simulink model "CML_Effort_Reward_Mapping"  (R2015a)
settings: Solver=ode4  SolverMode=MultiTasking  StartTime=0.0  StopTime=inf  FixedStep=BKIN_STEP_TIME  RelTol=1e-3
StartFcn:
  |  warndlg('Dexterit-E models cannot run under simulation. Please compile your model and run it from within Dexterit-E.');set_param(bdroot,'SimulationCommand','stop')
model workspace (MAT data in the model file):
  BKIN_STEP_TIME = 0.00025
  col_x = 1
  col_y = 2
  VRAD = 3
  COLOR = 4
  TARGET_COL = 2
  BKIN_KINEMATIC_FRAME_SIZE = 400
  E_NO_EVENT = 0
  K_START_TGT = 1
  INIT_DUR = 6
  TP_ITI = 10
  K_JOINT_ASSESSED = 2
  TEXT1 = 6
  TEXT2 = 7
  HEIGHT = 9
  STROKE_WIDTH = 10
  GOAL_F_PCT = 3
  DO_FDBK = 9
  MAX_MOVE_TIME = 8
  MIN_FORCE = 5
  E_TEST_MVC = 1
  E_HOLD_MVC = 3
  E_EOT = 10
  E_FORCE_TRIAL = 11
  E_HOLD_FORCE = 13
  K_BAR_TGT = 3
  K_MVC_TEXT_TGT = 5
  E_INIT_FORCE = 12
  E_SET_MVC = 2
  K_MVC = 6
  COLOR_SEL = 5
  ROTATION = 12
  K_RWD_TGT = 4
  E_ACCEPT_MVC = 5
  ACCEPT_MVC = 2
  REJECT_MVC = 3
  TEXT3 = 8
  REWARD_VAL = 4
  HOLD_TIME = 7
  E_REPORT_TRIAL = 21
  E_REPORT_RESPONSE = 22
  E_WAIT_JS_THRESH = 23
  E_AT_JS_THRESH = 24
  E_WAIT_JS = 27
  THEIGHT = 11
  TRIAL_TYPE = 1
  E_CHECK_MVC = 4
  E_REJECT_MVC = 6
  E_TRIAL_ACCEPTED = 25
  E_TRIAL_REJECTED = 26
undefined symbols (not defined in the file): magnitude
libraries: simulink x10, Video x9, slrtlib x8, General x3, KINARM_IO x2, KINARM_loads x2, KINARM_general x1, xpcnilib x1
(part 1 of 2)
CloseFcn:
  | rtwprivate ssgencode ModelCloseRequest b2lab2d
settings Model: ModifiedComment=chris -- Wed Feb 16 09:18:30 2005 -- Version 1.1384  ExtModeArmWhenConnect=off  ExtModeLogAll=off  LastModifiedBy=User
settings SolverCC: EnableConcurrentExecution=on  AutoInsertRateTranBlk=on
settings DataIOCC: LimitDataPoints=off  SignalLoggingSaveFormat=ModelDataLogs  SaveOutput=off  SaveTime=off  SignalLoggingName=sigsOut
settings OptimizationCC: BlockReduction=off  BooleanDataType=off  OptimizeBlockIOStorage=off  BufferReuse=off  GlobalBufferReuse=off  ExpressionFolding=off  ExpressionDepthLimit=2147483647  LocalBlockOutputs=off  InitFltsAndDblsToZero=on
settings DebuggingCC: SaveWithParameterizedLinksMsg=none  UnderspecifiedInitializationDetection=Classic  MergeDetectMultiDrivingBlocksExec=none  SignalResolutionControl=TryResolveAllWithWarning  MultiTaskDSMMsg=warning  FcnCallInpInsideContextMsg=UseLocalSettings  StateNameClashWarn=warning  StrictBusMsg=ErrorOnBusTreatedAsVector
settings HardwareCC: ProdIntDivRoundTo=Zero  ProdEndianess=LittleEndian  ProdLongLongMode=on  ProdHWDeviceType=Generic->32-bit x86 compatible  TargetHWDeviceType=32-bit Generic
settings SFSimCC: SimParseCustomCode=off
settings RTWCC: SystemTargetFile=slrt.tlc  TemplateMakefile=slrt_default_tmf  Description=Simulink Real-Time  RTWCompilerOptimization=on
settings CodeAppCC: MaxIdLength=63
settings SimulinkRealTimeCC: TargetFcnLib=ansi_tfl_tmw.mat  GeneratePreprocessorConditionals=Disable all  xPCisDownloadable=off

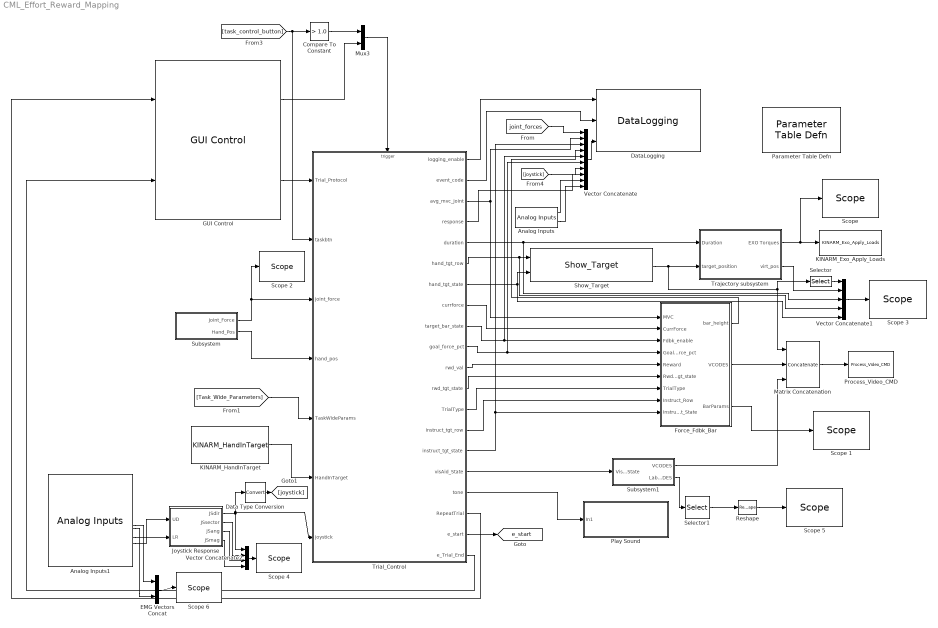
== system CML_Effort_Reward_Mapping ==
  Analog Inputs : KINARM_IO/Analog Inputs  channel=[18,19]  range=[5]  coupling=[0]  scantime6071e=1.28e-5  scantime6229=5e-6  sampletime=0.001  slot=-1  oscantime6071e=0
  Analog Inputs1 : KINARM_IO/Analog Inputs  channel=[1:32]  range=[5, 5, 5, 5, 5, 5, 5, 5,5, 5, 5, 5, 5, 5, 5, 5,5, 5, 5, 5, 5, 5, 5, 5,5, 5, 5, 5, 5, 5, 5, 5,]  coupling=[0, 0, 0, 0, 0, 0, 0, 0,0, 0, 0, 0, 0, 0, 0, 0,0, 0, 0, 0, 0, 0, 0, 0,0, 0, 0, 0, 0, 0, 0, 0,]  scantime6071e=1.28e-5  scantime6229=5e-6  sampletime=0.001  slot=-1  oscantime6071e=0
  Compare To Constant : simulink/Logic and Bit Operations/Compare To Constant  relop=>  const=1.0  OutDataTypeStr=boolean
  Data Type Conversion : DataTypeConversion
  DataLogging : General/DataLogging  log_event_codes=on  log_analog_inputs=on  show_time_remaining=off  ecat_include=on
      link override Poll KINARM/EPTorqueCMD: GotoTag=KINARMEPTorqueCMD
      link override Poll KINARM/TorqueCMD: GotoTag=KINARMTorqueCMD
  EMG Vectors Concat : Concatenate
  Force_Fdbk_Bar : Subsystem
  GUI Control : General/GUI Control  task_version=1.0  show_repeat_trial_flag=on  use_custom_tp=off  target_type_str=Circle  Target_Type=1  XYcols=[1 2]  Vcols=3  Lcols=4  indices_padding=[0 0 0 0;0 0 0 0]  target_table_rows=64  load_table_rows=20  tp_table_rows=100
  Joystick Response : Subsystem
  KINARM_Exo_Apply_Loads : KINARM_loads/KINARM_Exo_Apply_Loads  up_duration=1000  down_duration=1000  max_torque=10  limit_motors=off
  KINARM_HandInTarget : KINARM_general/KINARM_HandInTarget  use_dominant_hand=on  target_type=Circle  num_states=1  attribcol1=[VRAD]  attribcol2=[0]  attribcol3=[0]  attribcol4=[0]  attribcol5=[0]
  Matrix Concatenation : Concatenate  NumInputs=3  Mode=Multidimensional array
  Mux3 : Mux  Inputs=2
  Parameter Table Defn : General/Parameter Table Defn  ShowInLibBrowser=0
  Play Sound : Subsystem
  Process_Video_CMD : Video/Process_Video_CMD  video_delay=0
  Reshape : Reshape
  "Scope " : slrtlib/Displays and Logging/Scope   scopeno=6  scopetype=Target  autostart=on  viewmode=Numerical  formatstr='%15.6f'  grid=on  ylimits=[0,0]  nosamples=250  noprepostsamples=0  interleave=1  triggermode=FreeRun  triggersignal=1  trigsignalfromport=off  triggerlevel=0.0  triggerslope=Either  triggerscope=1  triggersample=0  filename=data.dat  mode=Lazy  writesize=512  autorestart=off  dynamicfilemode=off  maxwritefilesize=512*1024^2
  Scope 1 : slrtlib/Displays and Logging/Scope   scopeno=2  scopetype=Target  autostart=on  viewmode=Numerical  formatstr='%15.6f'  grid=on  ylimits=[0,0]  nosamples=250  noprepostsamples=0  interleave=1  triggermode=FreeRun  triggersignal=1  trigsignalfromport=off  triggerlevel=0.0  triggerslope=Either  triggerscope=1  triggersample=0  filename=data.dat  mode=Lazy  writesize=512  autorestart=off  dynamicfilemode=off  maxwritefilesize=512*1024^2
  Scope 2 : slrtlib/Displays and Logging/Scope   scopeno=3  scopetype=Target  autostart=on  viewmode=Numerical  formatstr='%15.6f'  grid=on  ylimits=[0,0]  nosamples=250  noprepostsamples=0  interleave=1  triggermode=FreeRun  triggersignal=1  trigsignalfromport=off  triggerlevel=0.0  triggerslope=Either  triggerscope=1  triggersample=0  filename=data.dat  mode=Lazy  writesize=512  autorestart=off  dynamicfilemode=off  maxwritefilesize=512*1024^2
  Scope 3 : slrtlib/Displays and Logging/Scope   scopeno=5  scopetype=Target  autostart=on  viewmode=Numerical  formatstr='%15.6f'  grid=on  ylimits=[0,0]  nosamples=250  noprepostsamples=0  interleave=1  triggermode=FreeRun  triggersignal=1  trigsignalfromport=off  triggerlevel=0.0  triggerslope=Either  triggerscope=1  triggersample=0  filename=data.dat  mode=Lazy  writesize=512  autorestart=off  dynamicfilemode=off  maxwritefilesize=512*1024^2
  Scope 4 : slrtlib/Displays and Logging/Scope   scopeno=1  scopetype=Target  autostart=on  viewmode=Numerical  formatstr='%15.6f'  grid=on  ylimits=[0,0]  nosamples=250  noprepostsamples=0  interleave=1  triggermode=FreeRun  triggersignal=1  trigsignalfromport=off  triggerlevel=0.0  triggerslope=Either  triggerscope=1  triggersample=0  filename=data.dat  mode=Lazy  writesize=512  autorestart=off  dynamicfilemode=off  maxwritefilesize=512*1024^2
  Scope 5 : slrtlib/Displays and Logging/Scope   scopeno=7  scopetype=Target  autostart=on  viewmode=Numerical  formatstr='%15.6f'  grid=on  ylimits=[0,0]  nosamples=250  noprepostsamples=0  interleave=1  triggermode=FreeRun  triggersignal=1  trigsignalfromport=off  triggerlevel=0.0  triggerslope=Either  triggerscope=1  triggersample=0  filename=data.dat  mode=Lazy  writesize=512  autorestart=off  dynamicfilemode=off  maxwritefilesize=512*1024^2
  Scope 6 : slrtlib/Displays and Logging/Scope   scopeno=8  scopetype=Target  autostart=on  viewmode=Numerical  formatstr='%15.6f'  grid=on  ylimits=[0,0]  nosamples=250  noprepostsamples=0  interleave=1  triggermode=FreeRun  triggersignal=1  trigsignalfromport=off  triggerlevel=0.0  triggerslope=Either  triggerscope=1  triggersample=0  filename=data.dat  mode=Lazy  writesize=512  autorestart=off  dynamicfilemode=off  maxwritefilesize=512*1024^2
  Selector : Selector  InputPortWidth=70  Indices=[3 4]
  Selector1 : Selector  NumberOfDimensions=2  InputPortWidth=3  IndexOptions=Index vector (dialog),Index vector (dialog)  Indices=[1],[1 2 3 4 15 65]  OutputSizes=1,1
  Show_Target : Video/Show_Target  target_type=Circle  num_states=1  attribcol1=[COLOR 0 0 VRAD]  attribcol2=[0 0 0 0]  attribcol3=[0 0 0 0]  attribcol4=[0 0 0 0]  attribcol5=[0 0 0 0]  stateindices_padding=[0 0 0 0 0 0 0;0 0 0 0 0 0 0;0 0 0 0 0 0 0;0 0 0 0 0 0 0;0 0 0 0 0 0 0]  source=dialog  opacity=100  target_display=Both subject and operator displays  num_col=4
  Subsystem : Subsystem
  Subsystem1 : Subsystem
  Trajectory subsystem : Subsystem
  Trial_Control : Stateflow chart  TreatAsAtomicUnit=on
  Vector Concatenate : Concatenate  NumInputs=10
  Vector Concatenate1 : Concatenate  NumInputs=5
  Vector Concatenate2 : Concatenate  NumInputs=4
  tag scope: e_start=global
  wires:
  Trial_Control/20(e_Trial_End) -> GUI Control/2
  GUI Control/1 -> Mux3/2
  Trial_Control/7(hand_tgt_state) -> Vector Concatenate1/5, Show_Target/2
  Trial_Control/6(hand_tgt_row) -> Vector Concatenate1/4, Show_Target/1
  Matrix Concatenation/1 -> Process_Video_CMD/1
  GUI Control/2 -> Trial_Control/1(Trial_Protocol)
  Trial_Control/1(logging_enable) -> DataLogging/1
  Trial_Control/19(e_start) -> [e_start]
  [joint_forces] -> Vector Concatenate/1
  Vector Concatenate/1 -> DataLogging/3
  Analog Inputs/1 -> Vector Concatenate/9
  Subsystem/1(Joint_Force) -> Scope 2/1, Trial_Control/3(joint_force)
  Subsystem/2(Hand_Pos) -> Trial_Control/4(hand_pos)
  [Task_Wide_Parameters] -> Trial_Control/5(TaskWideParams)
  Trial_Control/14(instruct_tgt_row) -> Force_Fdbk_Bar/8(Instruct_Row)
  Trial_Control/15(instruct_tgt_state) -> Vector Concatenate/3, Force_Fdbk_Bar/9(Instruct_State)
  Trial_Control/3(avg_mvc_joint) -> Force_Fdbk_Bar/1(MVC), Vector Concatenate/2
  Force_Fdbk_Bar/2(VCODES) -> Matrix Concatenation/2
  Force_Fdbk_Bar/1(bar_height) -> Vector Concatenate/4
  Force_Fdbk_Bar/3(BarParams) -> Scope 1/1
  Trial_Control/2(event_code) -> DataLogging/2
  Trial_Control/13(TrialType) -> Force_Fdbk_Bar/7(TrialType)
  KINARM_HandInTarget/1 -> Trial_Control/6(HandInTarget)
  Joystick Response/1(JSdir) -> Trial_Control/7(joystick), Data Type Conversion/1, Vector Concatenate2/1
  Analog Inputs1/24 -> Joystick Response/1(UD)
  Analog Inputs1/22 -> Joystick Response/2(LR)
  Data Type Conversion/1 -> [joystick]
  [joystick] -> Vector Concatenate/7
  Subsystem1/1(VCODES) -> Matrix Concatenation/3
  Trial_Control/11(rwd_val) -> Force_Fdbk_Bar/5(Reward)
  [task_control_button] -> Trial_Control/2(taskbtn), Compare To Constant/1
  Mux3/1 -> Trial_Control/Trigger
  Compare To Constant/1 -> Mux3/1
  Trial_Control/8(currforce) -> Force_Fdbk_Bar/2(CurrForce)
  Trial_Control/18(RepeatTrial) -> GUI Control/1
  Trial_Control/12(rwd_tgt_state) -> Force_Fdbk_Bar/6(Rwd_tgt_state)
  Trial_Control/17(tone) -> Play Sound/1(In1)
  Trial_Control/9(target_bar_state) -> Vector Concatenate/5, Force_Fdbk_Bar/3(Fdbk_enable)
  Trial_Control/10(goal_force_pct) -> Vector Concatenate/6, Force_Fdbk_Bar/4(Goal_force_pct)
  Trial_Control/4(response) -> Vector Concatenate/8
  Vector Concatenate1/1 -> Scope 3/1
  Selector/1 -> Vector Concatenate1/1
  Trajectory subsystem/2(virt_pos) -> Vector Concatenate1/2
  Show_Target/1 -> Matrix Concatenation/1, Selector/1, Trajectory subsystem/2(target_position)
  Trial_Control/5(duration) -> Vector Concatenate1/3, Trajectory subsystem/1(Duration)
  Trajectory subsystem/1(EXO Torques) -> "Scope "/1, KINARM_Exo_Apply_Loads/1
  Trial_Control/16(visAid_State) -> Subsystem1/1(VisAid_State)
  Vector Concatenate2/1 -> Scope 4/1
  Joystick Response/2(JSsector) -> Vector Concatenate2/2
  Joystick Response/3(JSang) -> Vector Concatenate2/3
  Joystick Response/4(JSmag) -> Vector Concatenate2/4
  Subsystem1/2(Label_VCODES) -> Selector1/1
  Selector1/1 -> Reshape/1
  Reshape/1 -> Scope 5/1
  EMG Vectors Concat/1 -> Scope 6/1
  Analog Inputs1/19 -> EMG Vectors Concat/2
  Analog Inputs1/18 -> EMG Vectors Concat/1
  Analog Inputs/2 -> Vector Concatenate/10

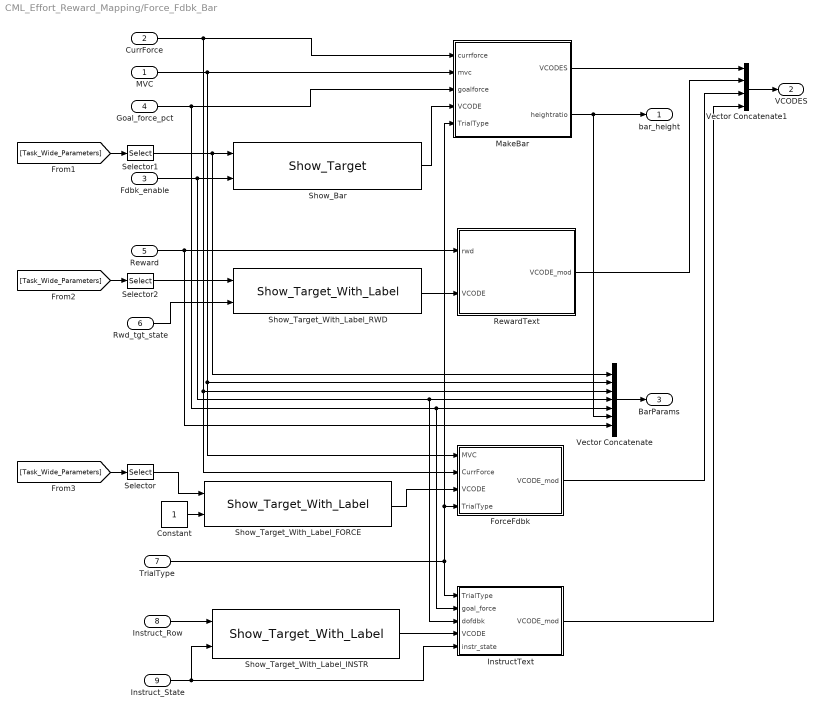
== system CML_Effort_Reward_Mapping/Force_Fdbk_Bar ==
  MVC : Inport
  CurrForce : Inport  Port=2
  Fdbk_enable : Inport  Port=3
  Goal_force_pct : Inport  Port=4
  Reward : Inport  Port=5
  Rwd_tgt_state : Inport  Port=6
  TrialType : Inport  Port=7
  Instruct_Row : Inport  Port=8
  Instruct_State : Inport  Port=9
  Constant : Constant
  ForceFdbk : MATLAB Function  TreatAsAtomicUnit=on
  InstructText : MATLAB Function  TreatAsAtomicUnit=on
  MakeBar : MATLAB Function  TreatAsAtomicUnit=on
  RewardText : MATLAB Function  TreatAsAtomicUnit=on
  Selector : Selector  InputPortWidth=50  Indices=[K_MVC_TEXT_TGT]
  Selector1 : Selector  InputPortWidth=50  Indices=[K_BAR_TGT]
  Selector2 : Selector  InputPortWidth=50  Indices=[K_RWD_TGT]
  Show_Bar : Video/Show_Target  target_type=Rectangle  num_states=1  attribcol1=[COLOR 0 STROKE_WIDTH VRAD HEIGHT 0]  attribcol2=[0 0 0 0 0 0]  attribcol3=[0 0 0 0 0 0]  attribcol4=[0 0 0 0 0 0]  attribcol5=[0 0 0 0 0 0]  stateindices_padding=[0 0 0 0 0;0 0 0 0 0;0 0 0 0 0;0 0 0 0 0;0 0 0 0 0]  source=dialog  opacity=100  target_display=Both subject and operator displays  num_col=6
  Show_Target_With_Label_FORCE : Video/Show_Target_With_Label  target_type=Rectangle  num_states=1  attribcol1=[0 0 0 VRAD HEIGHT 0 TEXT1 COLOR HEIGHT]  attribcol2=[0 0 0 0 0 0 0 0 0]  attribcol3=[0 0 0 0 0 0 0 0 0]  attribcol4=[0 0 0 0 0 0 0 0 0]  attribcol5=[0 0 0 0 0 0 0 0 0]  stateindices_padding=[0 0;0 0;0 0;0 0;0 0]  source=dialog  opacity=100  target_display=Operator display only
  Show_Target_With_Label_INSTR : Video/Show_Target_With_Label  target_type=Rectangle  num_states=3  attribcol1=[0 0 0 VRAD HEIGHT 0 TEXT1 COLOR HEIGHT]  attribcol2=[0 0 0 VRAD HEIGHT 0 TEXT2 COLOR HEIGHT]  attribcol3=[0 0 0 VRAD HEIGHT 0 TEXT3 COLOR HEIGHT]  attribcol4=[0 0 0 0 0 0 0 0 0]  attribcol5=[0 0 0 0 0 0 0 0 0]  stateindices_padding=[0 0;0 0;0 0;0 0;0 0]  source=dialog  opacity=100  target_display=Both subject and operator displays
  Show_Target_With_Label_RWD : Video/Show_Target_With_Label  target_type=Rectangle  num_states=1  attribcol1=[0 0 0 VRAD HEIGHT 0 TEXT1 COLOR HEIGHT]  attribcol2=[0 0 0 0 0 0 0 0 0]  attribcol3=[0 0 0 0 0 0 0 0 0]  attribcol4=[0 0 0 0 0 0 0 0 0]  attribcol5=[0 0 0 0 0 0 0 0 0]  stateindices_padding=[0 0;0 0;0 0;0 0;0 0]  source=dialog  opacity=100  target_display=Both subject and operator displays
  Vector Concatenate : Concatenate  NumInputs=7
  Vector Concatenate1 : Concatenate  NumInputs=4  Mode=Multidimensional array
  bar_height : Outport
  VCODES : Outport  Port=2
  BarParams : Outport  Port=3
  wires:
  Fdbk_enable/1 -> InstructText/3(dofdbk), Vector Concatenate/4, Show_Bar/2
  Selector1/1 -> Vector Concatenate/1, Show_Bar/1
  CurrForce/1 -> MakeBar/1(currforce), ForceFdbk/2(CurrForce), Vector Concatenate/3
  MVC/1 -> ForceFdbk/1(MVC), Vector Concatenate/2, MakeBar/2(mvc)
  Show_Bar/1 -> MakeBar/4(VCODE)
  MakeBar/1(VCODES) -> Vector Concatenate1/1
  Goal_force_pct/1 -> InstructText/2(goal_force), Vector Concatenate/5, MakeBar/3(goalforce)
  MakeBar/2(heightratio) -> Vector Concatenate/6, bar_height/1
  Vector Concatenate/1 -> BarParams/1
  Constant/1 -> Show_Target_With_Label_FORCE/2
  Show_Target_With_Label_FORCE/1 -> ForceFdbk/3(VCODE)
  ForceFdbk/1(VCODE_mod) -> Vector Concatenate1/3
  Vector Concatenate1/1 -> VCODES/1
  TrialType/1 -> InstructText/1(TrialType), MakeBar/5(TrialType), ForceFdbk/4(TrialType)
  Selector/1 -> Show_Target_With_Label_FORCE/1
  [Task_Wide_Parameters] -> Selector/1
  Show_Target_With_Label_INSTR/1 -> InstructText/4(VCODE)
  Instruct_Row/1 -> Show_Target_With_Label_INSTR/1
  Instruct_State/1 -> InstructText/5(instr_state), Show_Target_With_Label_INSTR/2
  InstructText/1(VCODE_mod) -> Vector Concatenate1/4
  [Task_Wide_Parameters] -> Selector1/1
  Selector2/1 -> Show_Target_With_Label_RWD/1
  [Task_Wide_Parameters] -> Selector2/1
  Show_Target_With_Label_RWD/1 -> RewardText/2(VCODE)
  RewardText/1(VCODE_mod) -> Vector Concatenate1/2
  Reward/1 -> RewardText/1(rwd), Vector Concatenate/7
  Rwd_tgt_state/1 -> Show_Target_With_Label_RWD/2

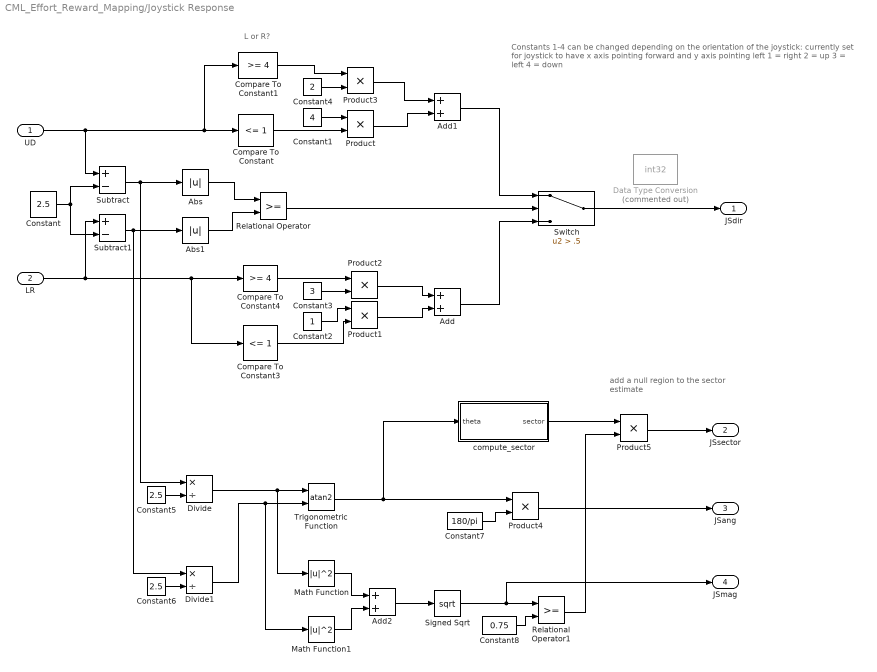
== system CML_Effort_Reward_Mapping/Joystick Response ==
  note: add a null region to the sector estimate
  note: Constants 1-4 can be changed depending on the orientation of the joystick:
      | currently set for joystick to have x axis pointing forward and y axis pointing left
      |
      | 1 = right
      | 2 = up
      | 3 = left
      | 4 = down
  note: L or R?
  UD : Inport
  LR : Inport  Port=2
  Abs : Abs
  Abs1 : Abs
  Add : Sum
  Add1 : Sum
  Add2 : Sum
  Compare To Constant : simulink/Logic and Bit Operations/Compare To Constant  relop=<=  const=1  OutDataTypeStr=boolean
  Compare To Constant1 : simulink/Logic and Bit Operations/Compare To Constant  relop=>=  const=4  OutDataTypeStr=boolean
  Compare To Constant3 : simulink/Logic and Bit Operations/Compare To Constant  relop=<=  const=1  OutDataTypeStr=boolean
  Compare To Constant4 : simulink/Logic and Bit Operations/Compare To Constant  relop=>=  const=4  OutDataTypeStr=boolean
  Constant : Constant  Value=2.5
  Constant1 : Constant  Value=4
  Constant2 : Constant
  Constant3 : Constant  Value=3
  Constant4 : Constant  Value=2
  Constant5 : Constant  Value=2.5
  Constant6 : Constant  Value=2.5
  Constant7 : Constant  Value=180/pi  VectorParams1D=off
  Constant8 : Constant  Value=0.75  VectorParams1D=off
  Data Type Conversion : DataTypeConversion  Commented=on  OutDataTypeStr=int32
  Divide : Product  Inputs=*/
  Divide1 : Product  Inputs=*/
  Math Function : Math  Operator=magnitude^2  SaturateOnIntegerOverflow=on
  Math Function1 : Math  Operator=magnitude^2  SaturateOnIntegerOverflow=on
  Product{,1..5} (6 alike) : Product
  Relational Operator : RelationalOperator  OutDataTypeStr=boolean
  Relational Operator1 : RelationalOperator  OutDataTypeStr=boolean
  Signed Sqrt : Sqrt  SaturateOnIntegerOverflow=on
  Subtract : Sum  Inputs=+-
  Subtract1 : Sum  Inputs=+-
  Switch : Switch  Criteria=u2 > Threshold  Threshold=.5
  Trigonometric Function : Trigonometry  Operator=atan2  OutputSignalType=real
  compute_sector : Subsystem
  JSdir : Outport
  JSsector : Outport  Port=2
  JSang : Outport  Port=3
  JSmag : Outport  Port=4
  wires:
  UD/1 -> Compare To Constant1/1, Compare To Constant/1, Subtract/1
  Compare To Constant/1 -> Product/2
  LR/1 -> Compare To Constant3/1, Compare To Constant4/1, Subtract1/1
  Compare To Constant3/1 -> Product1/2
  Compare To Constant4/1 -> Product2/1
  Subtract/1 -> Abs/1, Divide/1
  Subtract1/1 -> Divide1/1, Abs1/1
  Constant/1 -> Subtract/2, Subtract1/2
  Abs/1 -> Relational Operator/1
  Abs1/1 -> Relational Operator/2
  Compare To Constant1/1 -> Product3/1
  Constant1/1 -> Product/1
  Constant2/1 -> Product1/1
  Constant3/1 -> Product2/2
  Product2/1 -> Add/1
  Product1/1 -> Add/2
  Product/1 -> Add1/2
  Add1/1 -> Switch/1
  Add/1 -> Switch/3
  Relational Operator/1 -> Switch/2
  Constant4/1 -> Product3/2
  Product3/1 -> Add1/1
  Switch/1 -> JSdir/1
  Constant5/1 -> Divide/2
  Constant6/1 -> Divide1/2
  Divide/1 -> Math Function/1, Trigonometric Function/1
  Divide1/1 -> Math Function1/1, Trigonometric Function/2
  Trigonometric Function/1 -> Product4/1, compute_sector/1(theta)
  compute_sector/1(sector) -> Product5/1
  Math Function/1 -> Add2/1
  Math Function1/1 -> Add2/2
  Add2/1 -> Signed Sqrt/1
  Constant7/1 -> Product4/2
  Product4/1 -> JSang/1
  Relational Operator1/1 -> Product5/2
  Product5/1 -> JSsector/1
  Constant8/1 -> Relational Operator1/2
  Signed Sqrt/1 -> JSmag/1, Relational Operator1/1

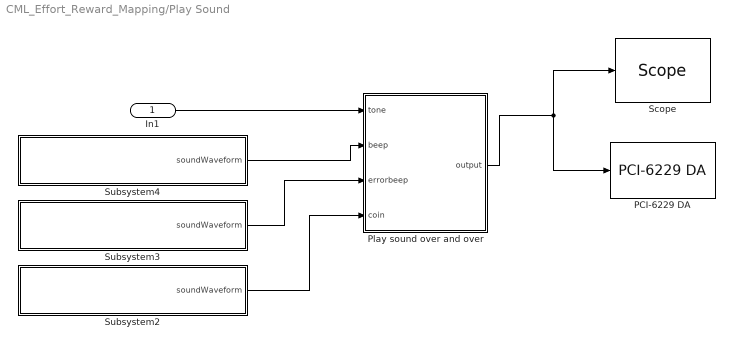
== system CML_Effort_Reward_Mapping/Play Sound ==
  In1 : Inport
  PCI-6229 DA : xpcnilib/D//A/M Series/PCI-6229 DA  channel=[1]  reset=[1]  initValue=[0]  sampletime=-1  slot=-1
  Play sound over and over : MATLAB Function  TreatAsAtomicUnit=on
  "Scope " : slrtlib/Displays and Logging/Scope   scopeno=4  scopetype=Target  autostart=on  viewmode=Graphical redraw  formatstr='%15.6f'  grid=on  ylimits=[0,0]  nosamples=4000  noprepostsamples=0  interleave=1  triggermode=FreeRun  triggersignal=1  trigsignalfromport=off  triggerlevel=0.0  triggerslope=Either  triggerscope=1  triggersample=0  filename=data.dat  mode=Lazy  writesize=512  autorestart=off  dynamicfilemode=off  maxwritefilesize=512*1024^2
  Subsystem2 : Subsystem  mask(Load Waveform Into Variable){fileName=coin.mat}
      mask prompts: fileName "Name of .mat Data File (must be in current directory)"
      mask help: This block will load the .MAT file specified in the dialog, and put the first variable into a GoTo called 'soundWaveform'.
      mask init:
      | filenameFromMask = get_param(gcb, 'fileName');
      | 
      | try 
      | 	dataFromFile = load(filenameFromMask);
      | 	names = fieldnames(dataFromFile);
      | 	soundDataFromFile = dataFromFile.(names{1});
      | 	display(['Sound waveform from file ''' filenameFromMask ''' loaded.']);
      | catch ME
      | 	display(ME.message)
      | end
      mask Help:
      | Enter the name a .MAT file containing a single vector or matrix. The .MAT file must be located in the current directory.
      | 
      | The first variable from the .MAT file will be put into a Goto called 'soundWaveform'.
      mask Display: disp(['Load waveform from ''' filenameFromMask ''''])
  Subsystem3 : Subsystem  mask(Load Waveform Into Variable){fileName=errorbeep.mat}
      mask prompts: fileName "Name of .mat Data File (must be in current directory)"
      mask help: This block will load the .MAT file specified in the dialog, and put the first variable into a GoTo called 'soundWaveform'.
      mask init: same as CML_Effort_Reward_Mapping/Play Sound/Subsystem2
      mask Help:
      | Enter the name a .MAT file containing a single vector or matrix. The .MAT file must be located in the current directory.
      | 
      | The first variable from the .MAT file will be put into a Goto called 'soundWaveform'.
      mask Display: disp(['Load waveform from ''' filenameFromMask ''''])
  Subsystem4 : Subsystem  mask(Load Waveform Into Variable){fileName=startbeep.mat}
      mask prompts: fileName "Name of .mat Data File (must be in current directory)"
      mask help: This block will load the .MAT file specified in the dialog, and put the first variable into a GoTo called 'soundWaveform'.
      mask init: same as CML_Effort_Reward_Mapping/Play Sound/Subsystem2
      mask Help:
      | Enter the name a .MAT file containing a single vector or matrix. The .MAT file must be located in the current directory.
      | 
      | The first variable from the .MAT file will be put into a Goto called 'soundWaveform'.
      mask Display: disp(['Load waveform from ''' filenameFromMask ''''])
  wires:
  Play sound over and over/1(output) -> PCI-6229 DA/1, "Scope "/1
  Subsystem3/1(soundWaveform) -> Play sound over and over/3(errorbeep)
  Subsystem4/1(soundWaveform) -> Play sound over and over/2(beep)
  In1/1 -> Play sound over and over/1(tone)
  Subsystem2/1(soundWaveform) -> Play sound over and over/4(coin)

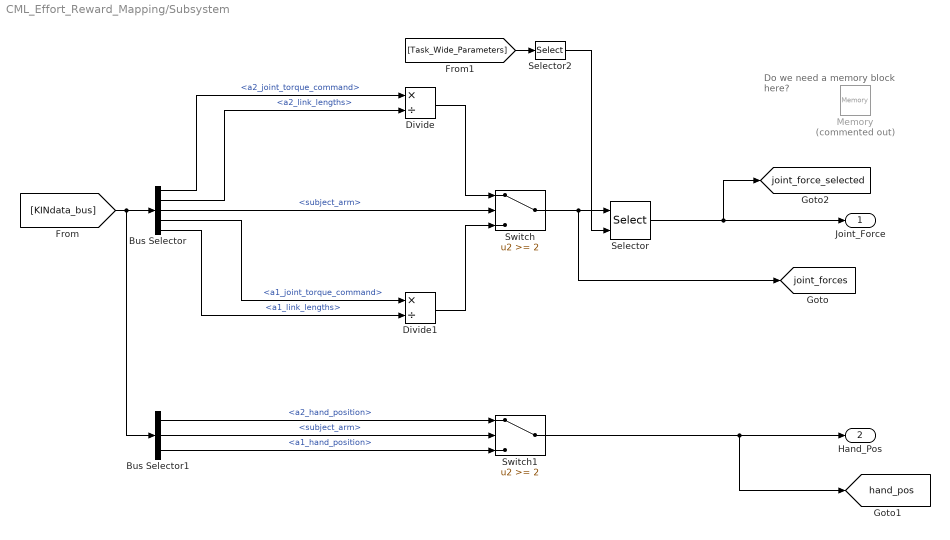
== system CML_Effort_Reward_Mapping/Subsystem ==
  note: Do we need a memory block here?
  Bus Selector : BusSelector  OutputSignals=Robot2.a2_joint_torque_command,Robot2.a2_link_lengths,KINDataGeneral.subject_arm,Robot1.a1_joint_torque_command,Robot1.a1_link_lengths
  Bus Selector1 : BusSelector  OutputSignals=Robot2.a2_hand_position,KINDataGeneral.subject_arm,Robot1.a1_hand_position
  Divide : Product  Inputs=*/
  Divide1 : Product  Inputs=*/
  Memory : Memory  Commented=on
  Selector : Selector  InputPortWidth=2  IndexOptions=Index vector (port)  Indices=[1 3]
  Selector2 : Selector  InputPortWidth=50  Indices=[K_JOINT_ASSESSED]
  Switch : Switch  Threshold=2
  Switch1 : Switch  Threshold=2
  Joint_Force : Outport
  Hand_Pos : Outport  Port=2
  tag scope: hand_pos=global, joint_force_selected=global, joint_forces=global
  wires:
  [KINdata_bus] -> Bus Selector1/1, Bus Selector/1
  Bus Selector/3 -> Switch/2  "<subject_arm>"
  Divide/1 -> Switch/1
  Divide1/1 -> Switch/3
  Bus Selector/1 -> Divide/1  "<a2_joint_torque_command>"
  Bus Selector/2 -> Divide/2  "<a2_link_lengths>"
  Bus Selector/4 -> Divide1/1  "<a1_joint_torque_command>"
  Bus Selector/5 -> Divide1/2  "<a1_link_lengths>"
  Bus Selector1/1 -> Switch1/1  "<a2_hand_position>"
  Bus Selector1/2 -> Switch1/2  "<subject_arm>"
  Bus Selector1/3 -> Switch1/3  "<a1_hand_position>"
  Switch/1 -> Selector/1, [joint_forces]
  Selector2/1 -> Selector/2
  Switch1/1 -> [hand_pos], Hand_Pos/1
  Selector/1 -> [joint_force_selected], Joint_Force/1
  [Task_Wide_Parameters] -> Selector2/1

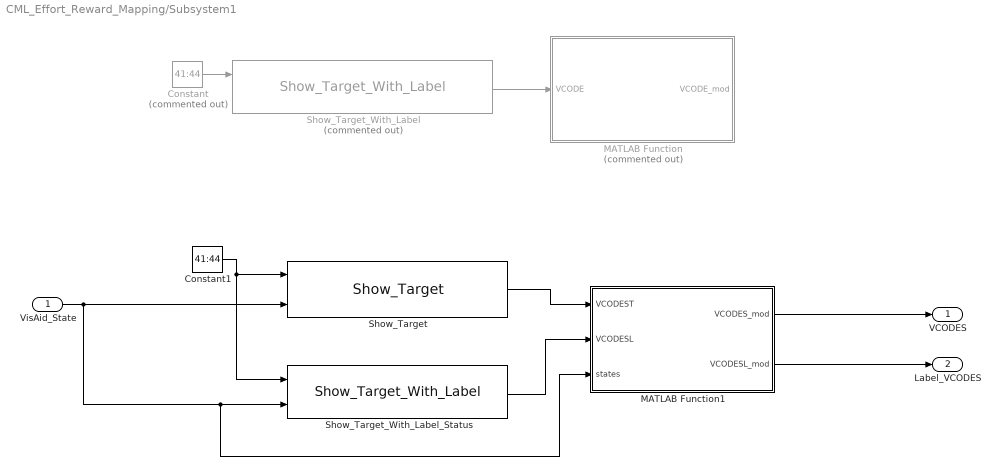
== system CML_Effort_Reward_Mapping/Subsystem1 ==
  VisAid_State : Inport
  Constant : Constant  Commented=on  Value=41:44
  Constant1 : Constant  Value=41:44
  MATLAB Function : MATLAB Function  Commented=on  TreatAsAtomicUnit=on
  MATLAB Function1 : MATLAB Function  TreatAsAtomicUnit=on
  Show_Target : Video/Show_Target  target_type=Triangle  num_states=2  attribcol1=[COLOR 0 0 VRAD THEIGHT 0 ROTATION]  attribcol2=[COLOR_SEL 0 0 VRAD THEIGHT 0 ROTATION]  attribcol3=[0 0 0 0 0 0 0]  attribcol4=[0 0 0 0 0 0 0]  attribcol5=[0 0 0 0 0 0 0]  stateindices_padding=[0 0 0 0;0 0 0 0;0 0 0 0;0 0 0 0;0 0 0 0]  source=dialog  opacity=100  target_display=Both subject and operator displays  num_col=7
  Show_Target_With_Label : Video/Show_Target_With_Label  Commented=on  target_type=Triangle  num_states=2  attribcol1=[COLOR 0 0 VRAD 0 0 ROTATION TEXT1 COLOR HEIGHT]  attribcol2=[COLOR_SEL 0 0 VRAD 0 0 ROTATION TEXT1 COLOR HEIGHT]  attribcol3=[0 0 0 0 0 0 0 0 0 0]  attribcol4=[0 0 0 0 0 0 0 0 0 0]  attribcol5=[0 0 0 0 0 0 0 0 0 0]  stateindices_padding=[0;0;0;0;0]  source=dialog  opacity=100  target_display=Both subject and operator displays
  Show_Target_With_Label_Status : Video/Show_Target_With_Label  target_type=Rectangle  num_states=2  attribcol1=[0 0 0 VRAD THEIGHT 0 TEXT1 COLOR HEIGHT]  attribcol2=[0 0 0 VRAD THEIGHT 0 TEXT1 COLOR HEIGHT]  attribcol3=[0 0 0 0 0 0 0 0 0]  attribcol4=[0 0 0 0 0 0 0 0 0]  attribcol5=[0 0 0 0 0 0 0 0 0]  stateindices_padding=[0 0;0 0;0 0;0 0;0 0]  source=dialog  opacity=100  target_display=Both subject and operator displays
  VCODES : Outport
  Label_VCODES : Outport  Port=2
  wires:
  Show_Target/1 -> MATLAB Function1/1(VCODEST)
  MATLAB Function1/1(VCODES_mod) -> VCODES/1
  ? -> Show_Target_With_Label/2
  Constant/1 -> Show_Target_With_Label/1
  Show_Target_With_Label/1 -> MATLAB Function/1(VCODE)
  Show_Target_With_Label_Status/1 -> MATLAB Function1/2(VCODESL)
  VisAid_State/1 -> MATLAB Function1/3(states), Show_Target_With_Label_Status/2, Show_Target/2
  MATLAB Function1/2(VCODESL_mod) -> Label_VCODES/1
  Constant1/1 -> Show_Target_With_Label_Status/1, Show_Target/1

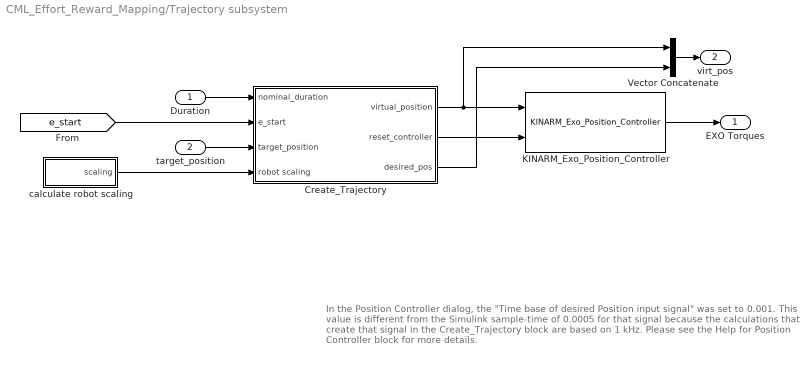
== system CML_Effort_Reward_Mapping/Trajectory subsystem ==
  note: In the Position Controller dialog, the "Time base of desired Position input signal" was set to 0.001.
      | This value is different from the Simulink sample-time of 0.0005 for that signal because the calculations
      | that create that signal in the Create_Trajectory block are based on 1 kHz. Please see the Help for
      | Position Controller block for more details.
  Duration : Inport
  target_position : Inport  Port=2
  Create_Trajectory : Subsystem
  KINARM_Exo_Position_Controller : KINARM_loads/KINARM_Exo_Position_Controller  use_dom_hand=on  KINARM_Type=Human  inertias_for_FF=KINARM robot  angles_or_XY=End-point (global x/y)  sample_time=0.001
  Vector Concatenate : Concatenate
  calculate robot scaling : Subsystem
  EXO Torques : Outport
  virt_pos : Outport  Port=2
  wires:
  Create_Trajectory/2(reset_controller) -> KINARM_Exo_Position_Controller/2
  Create_Trajectory/1(virtual_position) -> Vector Concatenate/1, KINARM_Exo_Position_Controller/1
  KINARM_Exo_Position_Controller/1 -> EXO Torques/1
  target_position/1 -> Create_Trajectory/3(target_position)
  Duration/1 -> Create_Trajectory/1(nominal_duration)
  [e_start] -> Create_Trajectory/2(e_start)
  calculate robot scaling/1(scaling) -> Create_Trajectory/4(robot scaling)
  Vector Concatenate/1 -> virt_pos/1
  Create_Trajectory/3(desired_pos) -> Vector Concatenate/2

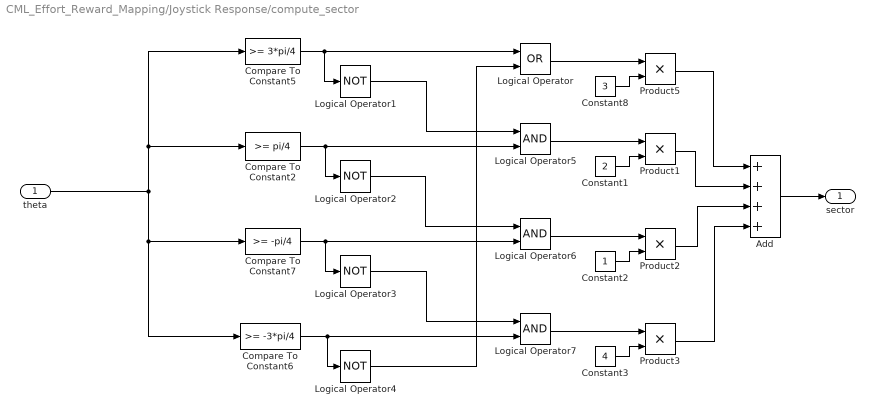
== system CML_Effort_Reward_Mapping/Joystick Response/compute_sector ==
  theta : Inport
  Add : Sum  Inputs=++++
  Compare To Constant2 : simulink/Logic and Bit Operations/Compare To Constant  relop=>=  const=pi/4  OutDataTypeStr=boolean
  Compare To Constant5 : simulink/Logic and Bit Operations/Compare To Constant  relop=>=  const=3*pi/4  OutDataTypeStr=boolean
  Compare To Constant6 : simulink/Logic and Bit Operations/Compare To Constant  relop=>=  const=-3*pi/4  OutDataTypeStr=boolean
  Compare To Constant7 : simulink/Logic and Bit Operations/Compare To Constant  relop=>=  const=-pi/4  OutDataTypeStr=boolean
  Constant1 : Constant  Value=2
  Constant2 : Constant
  Constant3 : Constant  Value=4
  Constant8 : Constant  Value=3
  Logical Operator : Logic  Operator=OR  AllPortsSameDT=off  OutDataTypeStr=boolean
  Logical Operator{1..4} (4 alike) : Logic  Operator=NOT  AllPortsSameDT=off  OutDataTypeStr=boolean
  Logical Operator5 : Logic  AllPortsSameDT=off  OutDataTypeStr=boolean
  Logical Operator6 : Logic  AllPortsSameDT=off  OutDataTypeStr=boolean
  Logical Operator7 : Logic  AllPortsSameDT=off  OutDataTypeStr=boolean
  Product{1..3,5} (4 alike) : Product
  sector : Outport
  wires:
  Logical Operator/1 -> Product5/1
  Constant8/1 -> Product5/2
  theta/1 -> Compare To Constant5/1, Compare To Constant2/1, Compare To Constant6/1, Compare To Constant7/1
  Compare To Constant5/1 -> Logical Operator1/1, Logical Operator/1
  Compare To Constant2/1 -> Logical Operator5/2, Logical Operator2/1
  Compare To Constant7/1 -> Logical Operator6/2, Logical Operator3/1
  Compare To Constant6/1 -> Logical Operator7/2, Logical Operator4/1
  Logical Operator4/1 -> Logical Operator/2
  Logical Operator1/1 -> Logical Operator5/1
  Logical Operator2/1 -> Logical Operator6/1
  Logical Operator3/1 -> Logical Operator7/1
  Logical Operator5/1 -> Product1/1
  Constant1/1 -> Product1/2
  Logical Operator6/1 -> Product2/1
  Constant2/1 -> Product2/2
  Logical Operator7/1 -> Product3/1
  Constant3/1 -> Product3/2
  Product5/1 -> Add/1
  Product1/1 -> Add/2
  Product2/1 -> Add/3
  Product3/1 -> Add/4
  Add/1 -> sector/1

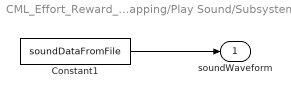
== system CML_Effort_Reward_Mapping/Play Sound/Subsystem2 ==
  Constant1 : Constant  Value=soundDataFromFile
  soundWaveform : Outport
  wires:
  Constant1/1 -> soundWaveform/1

== system CML_Effort_Reward_Mapping/Play Sound/Subsystem3 ==
  Constant1 : Constant  Value=soundDataFromFile
  soundWaveform : Outport
  wires:
  Constant1/1 -> soundWaveform/1

== system CML_Effort_Reward_Mapping/Play Sound/Subsystem4 ==
  Constant1 : Constant  Value=soundDataFromFile
  soundWaveform : Outport
  wires:
  Constant1/1 -> soundWaveform/1

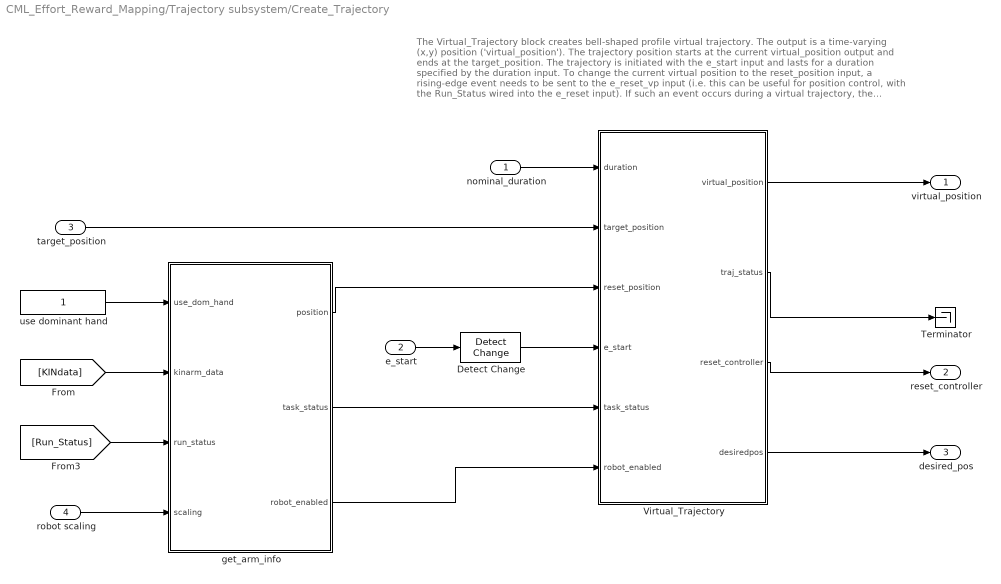
== system CML_Effort_Reward_Mapping/Trajectory subsystem/Create_Trajectory ==
  note: The Virtual_Trajectory block creates bell-shaped profile virtual trajectory.
      | The output is a time-varying (x,y) position ('virtual_position').
      |
      | The trajectory position starts at the current virtual_position output and ends at the target_position.
      | The trajectory is initiated with the e_start input and lasts for a duration specified by the duration input.
      |
      | To change the current virtual position to the reset_position input, a rising-edge event needs to be sent to the e_reset_vp input
      | (i.e. this can be useful for position control, with the Run_Status wired into the e_reset input).
      | If such an event occurs during a virtual trajectory, the trajectory is halted immediately.
  nominal_duration : Inport
  e_start : Inport  Port=2
  target_position : Inport  Port=3
  robot scaling : Inport  Port=4
  Detect Change : simulink/Logic and Bit Operations/Detect Change  vinit=0  InputProcessing=Inherited  OutDataTypeStr=uint8
  Terminator : Terminator
  Virtual_Trajectory : Subsystem
  get_arm_info : MATLAB Function  TreatAsAtomicUnit=on
  use dominant hand : Constant
  virtual_position : Outport
  reset_controller : Outport  Port=2
  desired_pos : Outport  Port=3
  wires:
  Virtual_Trajectory/1(virtual_position) -> virtual_position/1
  nominal_duration/1 -> Virtual_Trajectory/1(duration)
  e_start/1 -> Detect Change/1
  target_position/1 -> Virtual_Trajectory/2(target_position)
  Detect Change/1 -> Virtual_Trajectory/4(e_start)
  use dominant hand/1 -> get_arm_info/1(use_dom_hand)
  [KINdata] -> get_arm_info/2(kinarm_data)
  get_arm_info/1(position) -> Virtual_Trajectory/3(reset_position)
  Virtual_Trajectory/3(reset_controller) -> reset_controller/1
  get_arm_info/2(task_status) -> Virtual_Trajectory/5(task_status)
  get_arm_info/3(robot_enabled) -> Virtual_Trajectory/6(robot_enabled)
  [Run_Status] -> get_arm_info/3(run_status)
  Virtual_Trajectory/2(traj_status) -> Terminator/1
  robot scaling/1 -> get_arm_info/4(scaling)
  Virtual_Trajectory/4(desiredpos) -> desired_pos/1

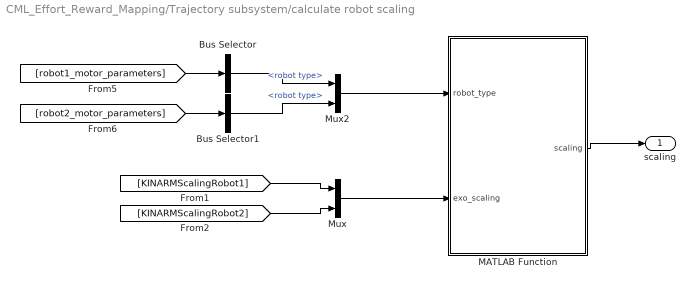
== system CML_Effort_Reward_Mapping/Trajectory subsystem/calculate robot scaling ==
  Bus Selector : BusSelector  OutputSignals=robot type
  Bus Selector1 : BusSelector  OutputSignals=robot type
  MATLAB Function : MATLAB Function  TreatAsAtomicUnit=on
  Mux : Mux  Inputs=2
  Mux2 : Mux  Inputs=2
  scaling : Outport
  wires:
  [KINARMScalingRobot1] -> Mux/1
  [KINARMScalingRobot2] -> Mux/2
  Mux/1 -> MATLAB Function/2(exo_scaling)
  Mux2/1 -> MATLAB Function/1(robot_type)
  MATLAB Function/1(scaling) -> scaling/1
  [robot2_motor_parameters] -> Bus Selector1/1
  Bus Selector1/1 -> Mux2/2  "<robot type>"
  Bus Selector/1 -> Mux2/1  "<robot type>"
  [robot1_motor_parameters] -> Bus Selector/1

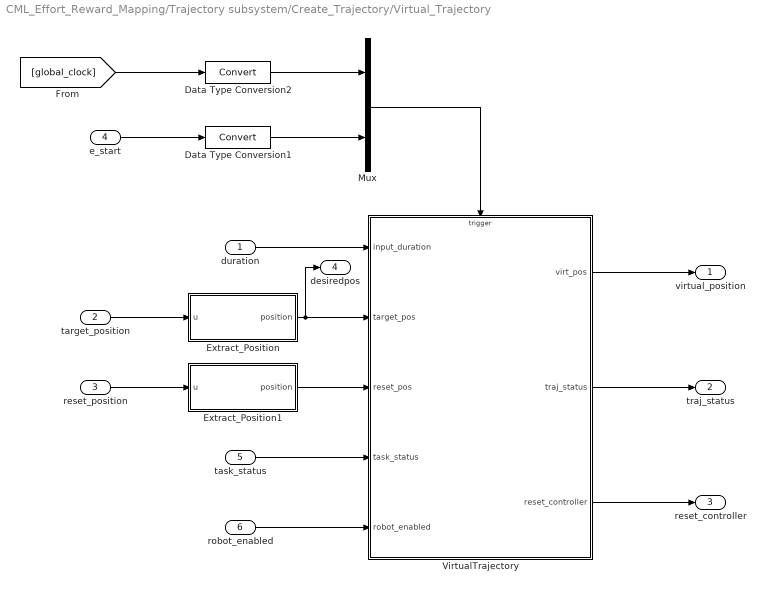
== system CML_Effort_Reward_Mapping/Trajectory subsystem/Create_Trajectory/Virtual_Trajectory ==
  duration : Inport
  target_position : Inport  Port=2
  reset_position : Inport  Port=3
  e_start : Inport  Port=4
  task_status : Inport  Port=5
  robot_enabled : Inport  Port=6
  Data Type Conversion1 : DataTypeConversion
  Data Type Conversion2 : DataTypeConversion
  Extract_Position : MATLAB Function  TreatAsAtomicUnit=on
  Extract_Position1 : MATLAB Function  TreatAsAtomicUnit=on
  Mux : Mux  Inputs=2
  VirtualTrajectory : Stateflow chart  TreatAsAtomicUnit=on
  virtual_position : Outport
  traj_status : Outport  Port=2
  reset_controller : Outport  Port=3
  desiredpos : Outport  Port=4
  wires:
  e_start/1 -> Data Type Conversion1/1
  target_position/1 -> Extract_Position/1(u)
  [global_clock] -> Data Type Conversion2/1
  Mux/1 -> VirtualTrajectory/Trigger
  duration/1 -> VirtualTrajectory/1(input_duration)
  VirtualTrajectory/1(virt_pos) -> virtual_position/1
  Extract_Position/1(position) -> desiredpos/1, VirtualTrajectory/2(target_pos)
  reset_position/1 -> Extract_Position1/1(u)
  Data Type Conversion2/1 -> Mux/1
  VirtualTrajectory/2(traj_status) -> traj_status/1
  robot_enabled/1 -> VirtualTrajectory/5(robot_enabled)
  task_status/1 -> VirtualTrajectory/4(task_status)
  Data Type Conversion1/1 -> Mux/2
  Extract_Position1/1(position) -> VirtualTrajectory/3(reset_pos)
  VirtualTrajectory/3(reset_controller) -> reset_controller/1

== stateflow chart CML_Effort_Reward_Mapping/Trial_Control ==
  settings: sampleTime=0.001
  state init/
    //bring the hand to the start position
    mvc_joint = 0;
    avg_mvc_joint = TaskWideParams[K_MVC];
    n_mvc = 1*(avg_mvc_joint > 1e-4); //if initial MVC is nonzero, add 1
    hand_tgt_row = TaskWideParams[K_START_TGT];
    hand_tgt_state = 1;
    instruct_tgt_row = 0;
    instruct_tgt_state = 0;
    AcceptTrials = 0; //not sure if we can initialize a whole array like this?
    duration = 2000;
  state Main_Trial
    state InitApplyTrial/
      event_code = E_FORCE_TRIAL;
      logging_enable = 1;
      instruct_tgt_row = Trial_Protocol[TARGET_COL];
      instruct_tgt_state = 1;
      tmpforce = 0;
      tmpcounter = 0;
      iforce = 0;
      maxforce = 0;
      [Itrial,TestedTrials,Ntested] = trialselect(Ntrials,TestedTrials,Ntested);
      goal_force_pct = AcceptTrials[Itrial][1];
      goal_force = avg_mvc_joint*(goal_force_pct/100.0);
      target_bar_state = 1;
      rwd_val = AcceptTrials[Itrial][2];
      rwd_tgt_state = 1;
      min_force = Trial_Protocol[MIN_FORCE];
      force_thresh = min_force;
      force_thresh += force_thresh*(target_bar_state == 0); //if no feedback, relax the criterion
      hold_time = Trial_Protocol[HOLD_TIME];
      max_move_time = Trial_Protocol[MAX_MOVE_TIME];
      tone = 1;
      tick = 0;
    state InitMVC/
      event_code = E_TEST_MVC;
      logging_enable = 1;
      duration = 1;
      instruct_tgt_row = Trial_Protocol[TARGET_COL];
      instruct_tgt_state = 1;
      target_bar_state = 0;
      min_force = Trial_Protocol[MIN_FORCE];
      tmpforce = 0;
      maxforce = min_force;
      currforce = 0;
      hold_time = Trial_Protocol[HOLD_TIME];
      max_move_time = Trial_Protocol[MAX_MOVE_TIME];
      tick = 0;
      tone = 1;
      currforce = 0;
    state InitReportTrial/
      event_code = E_REPORT_TRIAL;
      logging_enable = 1;
      instruct_tgt_row = Trial_Protocol[TARGET_COL];
      instruct_tgt_state = 1;
      goal_force_pct = Trial_Protocol[GOAL_F_PCT];
      goal_force = avg_mvc_joint*(goal_force_pct/100.0);
      target_bar_state = 1;
      rwd_val = Trial_Protocol[REWARD_VAL];
      rwd_tgt_state = 1;
      hold_time = Trial_Protocol[HOLD_TIME];
    state WaitResponse/ [commented out]
      event_code = E_REPORT_RESPONSE;
      resp_tgt_state = 1;
      tone = 1;
    state SetMVC/
      event_code = E_SET_MVC;
      tmpcounter = 0;
      tmp_forcehist = 0;
      iforce = 0;
      during: //check and update the estimated mvc
      tick++;
      currforce = joint_force;
      [maxforce,iforce,tmp_forcehist] = calcmvc(tmp_forcehist,iforce,joint_force)
    state HoldMVC/
      event_code = E_HOLD_MVC;
      tone = 0;
      during: //check and update the estimated mvc
      tick++;
      tmpcounter++;
      currforce = joint_force;
    state ApplyForce/
      event_code = E_INIT_FORCE;
      during:
      maxforce = joint_force;
      currforce = joint_force;
      tmpcounter = 0;
      tick++;
    state WaitForThreshold/
      event_code = E_WAIT_JS_THRESH;
      visAid_State[1] =1; visAid_State[2] =0;
      visAid_State[3] =1; visAid_State[4] =0;
      response = joystick;
      during:
      response = joystick;
    state TimeAtThresh/
      event_code = E_AT_JS_THRESH;
      hold_time = 300;
    state WaitAcceptMVC/
      event_code = E_CHECK_MVC;
      currforce = maxforce;
      instruct_tgt_state = 2;
      tone = 1;
    state HoldAppliedForce/
      event_code = E_HOLD_FORCE;
      during:
      maxforce = joint_force;
      currforce = joint_force;
      tmpcounter++;
      tick++;
    state HoldReject/
      instruct_tgt_state = 3;
      event_code = E_TRIAL_REJECTED;
    state AcceptMVC/
      event_code = E_ACCEPT_MVC;
      //record the MVC on this trial if desired
      mvc_joint += maxforce; %*(tmpcounter >= force_hold_time);
      n_mvc += 1; %*(tmpcounter >= force_hold_time);
      avg_mvc_joint = mvc_joint/n_mvc;
    state EndMVC/
      event_code = E_EOT;
    state Success/
      instruct_tgt_state = 2;
      tone = 2;
      hold_time = 800;
    state RememberAccept/
      //log accept trials
      event_code = E_TRIAL_ACCEPTED;
      instruct_tgt_state = 2;
      [AcceptTrials,Ntrials] = savetrial(AcceptTrials,Ntrials,goal_force_pct,rwd_val)
    state Failure/
      instruct_tgt_state = 3;
      tone = 3;
      hold_time = 1200;
    state EndOfResponseTrial/
      event_code = E_EOT;
      //instruct_tgt_state = 0;
      target_bar_state = 0;
      rwd_tgt_state = 0;
      visAid_State[response] = 0;
    state ResetJoystick/
      event_code = E_WAIT_JS;
    state EndOfTrial/
      event_code = E_EOT;
      //instruct_tgt_state = 2;
    (junction 75) -> InitMVC [order 3] : [after(duration, e_clk)  && (TrialType == 1)]
    (junction 75) -> InitApplyTrial [order 1] : [after(duration, e_clk) && (TrialType == 3)]
    (junction 75) -> InitReportTrial [order 2] : [TrialType == 2]
    InitReportTrial -> WaitForThreshold : after(hold_time,e_clk)
    InitReportTrial -> WaitResponse [commented out] : after(hold_time,e_clk)
    InitMVC -> SetMVC : [(joint_force > min_force) && after(1, e_clk)]/
    WaitResponse -> WaitForThreshold [commented out] : after(100,e_clk)
    InitApplyTrial -> ApplyForce : [(joint_force > min_force) && after(1, e_clk)]
    SetMVC -> HoldMVC [order 1] : [abs(joint_force - maxforce) < min_force]
    HoldMVC -> SetMVC [order 2] : [abs(joint_force-maxforce) > min_force]
    ApplyForce -> Failure [order 1] : [tick > max_move_time]
    HoldMVC -> WaitAcceptMVC [order 1] : [(tmpcounter >= hold_time)]
    SetMVC -> WaitAcceptMVC [order 2] : [(tick > max_move_time) ]
    WaitForThreshold -> TimeAtThresh : [after(1,e_clk) && (response == 1 || response == 3)]/
        | visAid_State[response] = 2;
        | //only happens if past thresh
    TimeAtThresh -> WaitForThreshold [order 2] : [after(1,e_clk) && (joystick < 1  || response ~= joystick)]/
        | visAid_State[response] = 1;
        | response = 0;
    ApplyForce -> HoldAppliedForce [order 2] : [abs(joint_force - goal_force) < force_thresh]
    HoldAppliedForce -> ApplyForce [order 1] : [abs(joint_force - goal_force) > force_thresh]/
        | //apply the force threshold on either side of the goal
    TimeAtThresh -> (junction 163) [order 1] : [after(hold_time,e_clk)]/
        | visAid_State[1] =0; visAid_State[2] =0;
        | visAid_State[3] =0; visAid_State[4] =0;
        | visAid_State[response] = 2;
    WaitAcceptMVC -> AcceptMVC [order 1] : [taskbtn == 2]
    WaitAcceptMVC -> EndMVC [order 2] : [taskbtn == 3]/
        | RepeatTrial = 1;
        | event_code = E_REJECT_MVC;
    (junction 163) -> HoldReject [order 2] : [response == 3]/
    (junction 163) -> RememberAccept [order 1] : [response == 1]/
    HoldReject -> EndOfResponseTrial : after(500,e_clk)
    HoldAppliedForce -> Success [order 3] : [tmpcounter > hold_time]
    HoldAppliedForce -> Failure [order 2] : [tick > max_move_time]
    AcceptMVC -> EndMVC
    EndOfResponseTrial -> ResetJoystick [order 1] : [joystick > 0]
    RememberAccept -> EndOfResponseTrial : after(500,e_clk)
    EndOfResponseTrial -> (junction 220) [order 2]
    Failure -> EndOfTrial : after(hold_time,e_clk)
    Success -> EndOfTrial : after(hold_time,e_clk)
    EndMVC -> (junction 111) : [joint_force <= min_force]
    ResetJoystick -> (junction 220) : [joystick == 0]
    (junction 220) -> (junction 111)
    EndOfTrial -> (junction 111) : [joint_force <= min_force]
  state MovToStart/
    ITI = Trial_Protocol[TP_ITI];
    TrialType = Trial_Protocol[TRIAL_TYPE];
    RepeatTrial = 0;
    instruct_tgt_state = 0;
    rwd_tgt_state = 0;
    target_bar_state = 0;
    tone = 0;
    currforce = 0;
    e_start;
  state Inter_Trial_State/
    e_Trial_End
    duration = Trial_Protocol[INIT_DUR];
    instruct_tgt_state = 0;
    hand_tgt_state = 0;
  state WaitForFlagToSet
  (default) -> init
  init -> (junction 85)
  MovToStart -> (junction 75) : [HandInTarget[hand_tgt_row]]/
      | //hand_tgt_state = 0;
  (junction 85) -> MovToStart
  Inter_Trial_State -> (junction 85)
  WaitForFlagToSet -> Inter_Trial_State : after(2, e_clk)
  Main_Trial -> WaitForFlagToSet : e_ExitTrialNow/
      | instruct_tgt_state = 0;
      | hand_tgt_state = 0;
      | logging_enable = 0;
      | tickCount = 10;
  (junction 111) -> Inter_Trial_State : after(ITI, e_clk)
  data: forcehist function_input double size=[200,1]; itrial function_input double; meanmvc function_output double; itrial1 function_output double; force function_input double; forcehist1 function_output double size=[200,1]; ntrials function_input double; testedtrials function_input double size=[100,1]; itrial function_output double; ntested function_input double; tested function_output double size=[100,1]; ntest function_output double; trialtable function_input double size=[100,2]; ntrials function_input double; force function_input double; rwd function_input double; trials function_output double size=[100,2]; ntrials1 function_output double; logging_enable output boolean; event_code output double; avg_mvc_joint output double; response output double; mvc_joint local double; duration output double; hand_tgt_row output [1..32]; hand_tgt_state output double; currforce output double; tickCount local double; Trial_Protocol input double; taskbtn input double; max_move_time local double size=1; joint_force input double; target_bar_state output double; goal_force_pct output double; rwd_val output double; rwd_tgt_state output double; TrialType output double; hand_pos input double size=2; TaskWideParams input double size=50; instruct_tgt_row output double; instruct_tgt_state output double; n_mvc local double; tmp_forcehist local double size=[200,1] =0; tmp_counter local double; iforce local double; hold_time local double; goal_force local double; maxforce local double; min_force local double; tick local double; tmpcounter local double; tmpforce local double; ITI local double; HandInTarget input double; force_thresh local double; joystick input double; visAid_State output double size=4; Ntrials local double; AcceptTrials local double size=[100,2] =0; TestedTrials local double size=[100,1]; Ntested local double; tone output double; RepeatTrial output double; Itrial local double
  data hand_tgt_row settings: description=index of the row currently being used in the TargetTable
  events: e_btn input EITHER_EDGE_EVENT; e_start output EITHER_EDGE_EVENT; e_clk input RISING_EDGE_EVENT; e_ExitTrialNow input EITHER_EDGE_EVENT; e_Trial_End output EITHER_EDGE_EVENT
  function [meanmvc,itrial1,forcehist1] = calcmvc(forcehist,itrial,force):
    | function [meanmvc,itrial1,forcehist1] = calcmvc(forcehist,itrial,force)
    |  
    |  
    | itrial1 = itrial+1;
    | if itrial1 > length(forcehist)
    |     itrial1 = 1;
    | end
    | 
    | forcehist(itrial1) = force;
    | 
    | meanmvc = sum(forcehist)/sum(forcehist>0);
    | 
    | %meanmvc = mean(nonzeros(forcehist));
    | 
    | forcehist1 = forcehist;
  function [itrial,tested,ntest] = trialselect(ntrials,testedtrials,ntested):
    | function [itrial,tested,ntest] = trialselect(ntrials,testedtrials,ntested)
    |  
    | ntested = ntested+1;
    | 
    | alltrials = zeros(size(testedtrials));
    | 
    | itrial = 0;
    | %alltrials(1:ntrials) = 1:ntrials; %make a vector of all possible trials
    | %alltrials(ntrials+1:end) = 0;
    | 
    | %initialize a vector of all trials
    | alltrials = [1:100]';
    | 
    | %set all extra and previously tested trials to zero
    | for i = ntrials+1:100
    |     alltrials(i) = 0;
    | end
    | for i = 1:ntrials
    |     alltrials(testedtrials(i)) = 0; %remove the ones we already tested
    | end
    | 
    | alltrials = sort(alltrials,'descend'); %put all the zeros at the end
    | ntrials = ntrials-sum(testedtrials>0); %number of valid trials
    | 
    | %alltrials = setdiff( alltrials,testedtrials(1:(ntested-1)) ); %remove the ones we already tested
    | 
    | %alltrials = alltrials(randperm(length(alltrials))); %shuffle the remaining vector
    | %itrial = alltrials(1); %pull the first element as the new trial
    | 
    | itrial = round(rand*(ntrials-1))+1;
    | 
    | itrial = alltrials(itrial);
    | 
    | testedtrials(ntested) = itrial; %record which trial we will be testing
    | 
    | %set the outputs
    | tested = testedtrials;
    | ntest = ntested;
  function [trials,ntrials1]  = savetrial(trialtable,ntrials,force,rwd):
    | function [trials,ntrials1]  = savetrial(trialtable,ntrials,force,rwd)
    |  
    | ntrials = ntrials+1;
    | 
    | trialtable(ntrials,:) = [force, rwd];
    | 
    | trials = trialtable;
    | ntrials1 = ntrials;

== matlab function CML_Effort_Reward_Mapping/Trajectory subsystem/calculate robot scaling/MATLAB Function ==
  data: robot_type input; scaling output; exo_scaling input
function scaling = fcn(robot_type, exo_scaling)
%#codegen

scaling = [0, 0];

%0 = EXO, 1 = EP, 2 = NHP
for n=1:2
    if robot_type(n) == 1
        scaling(n) = 0;
    else
        scaling(n) = exo_scaling(n);
    end
end

== matlab function CML_Effort_Reward_Mapping/Trajectory subsystem/Create_Trajectory/Virtual_Trajectory/Extract_Position ==
  settings: fimath=|
      | fimath(...
      | 'RoundMode', 'floor',...
      | 'OverflowMode', 'wrap',...
      | 'ProductMode', 'KeepLSB', 'ProductWordLength', 32,...
      | 'SumMode', 'KeepLSB', 'SumWordLength', 32,...
      | 'CastBeforeSum', false)
  data: u input; position output
function position = fcn(u)

position=[0,0];	%initialization
if length(u)==2	%input is assumed to be (x,y) position, global coordinates, (m)		
	position=u;
else			%input is assumed to be a VCODE
	position(1)=u(3);
	position(2)=u(4);
end

== matlab function CML_Effort_Reward_Mapping/Trajectory subsystem/Create_Trajectory/Virtual_Trajectory/Extract_Position1 ==
  settings: fimath=|
      | fimath(...
      | 'RoundMode', 'floor',...
      | 'OverflowMode', 'wrap',...
      | 'ProductMode', 'KeepLSB', 'ProductWordLength', 32,...
      | 'SumMode', 'KeepLSB', 'SumWordLength', 32,...
      | 'CastBeforeSum', false)
  data: u input; position output
function position = fcn(u)

position=[0,0];	%initialization
if length(u)==2	%input is assumed to be (x,y) position, global coordinates, (m)		
	position=u;
else			%input is assumed to be a VCODE
	position(1)=u(3);
	position(2)=u(4);
end
